simulink model "uz_mlp_three_layer"  (R2021a)
settings: Solver=FixedStepDiscrete  StartTime=0.0  StopTime=5000  RelTol=1e-3
values from neighbouring files (symbols this model uses):
  nn = nn.set_all_parameter(rand_variables)    [mlp2_definition.m]
  nn_data_type_max = 131071    [mlp2_definition.m]
  numInput = 13    [mlp2_definition.m]
  numOut = 4    [mlp2_definition.m]
libraries: hdlsllib x90, simulink x79, el_machinelearning x2
(part 3 of 4)

== system uz_mlp_three_layer/uz_mlp_three_layer/reluLayer_8Parallel/MAC7 ==
  rd_addr : Inport
  b : Inport  Port=2
  axi_signals : Inport  Port=3
  fromStateMachine : Inport  Port=4
  AND : Logic  IconShape=distinctive  AllPortsSameDT=off  OutDataTypeStr=boolean
  AND1 : Logic  IconShape=distinctive  AllPortsSameDT=off  OutDataTypeStr=boolean
  Bus Selector : BusSelector  OutputSignals=axi_weightData,axi_weightAddr,axi_weightsWriteEnable,axi_biasData,axi_biasAddr,axi_biasWriteEnable,axi_layerNr
  Bus Selector1 : BusSelector  OutputSignals=endin,validIn,startin,mac_counter,write_enable,n_perceptron
  Compare To Constant : simulink/Logic and Bit Operations/Compare To Constant  relop===  const=ParallelNr  OutDataTypeStr=boolean
  Compare To Constant1 : simulink/Logic and Bit Operations/Compare To Constant  relop===  const=ParallelNr  OutDataTypeStr=boolean
  Compare To Constant2 : simulink/Logic and Bit Operations/Compare To Constant  relop===  const=LayerNr  OutDataTypeStr=boolean
  Constant : Constant  Value=nStart  OutDataTypeStr=Inherit: Inherit via back propagation  SampleTime=-1
  Dual Port RAM System1 : hdlsllib/HDL RAMs/Dual Port RAM System  RAMType=Simple dual port  WriteOutputValue=New data  RAMInitialValue=[layer.bias(nStart:nEnd);zeros(1024-length(layer.bias(nStart:nEnd)),1)]  SimulateUsing=Code generation
      settings: SourceProductBaseCode=SL
  Dual Port RAM System2 : hdlsllib/HDL RAMs/Dual Port RAM System  RAMType=Simple dual port  WriteOutputValue=New data  RAMInitialValue=[0]  SimulateUsing=Code generation
      settings: SourceProductBaseCode=SL
  Dual Port RAM System3 : hdlsllib/HDL RAMs/Dual Port RAM System  RAMType=Simple dual port  WriteOutputValue=New data  RAMInitialValue=[0;reshape(layer.weights(:,nStart:nEnd),[],1);zeros(1023-length(reshape(layer.weights(:,nStart:nEnd),[],1)),1)]  SimulateUsing=Code generation
      settings: SourceProductBaseCode=SL
  Gain : Gain  Gain=size(layer.weights(:,nStart:nEnd),1)  OutDataTypeStr=Inherit: Same as input
  Multiply-Accumulate1 : hdlsllib/HDL Operations/Multiply-Accumulate  opMode=Streaming - using Start and End ports  initValueSetting=Dialog  initValue=0  initValueSetting2=Input port  initValue2=0  initValueSetting3=Dialog  initValue3=0  num_samples=2  RndMeth2=Floor  RndMeth3=Floor  datatype2=fixdt(1,32,14)  datatype3=Inherit: Inherit via back propagation  validOut=on  endInandOut=on  startOut=on  countOut=on  dim=-1  DoSatur=off  parallel=off
      settings: SourceProductBaseCode=SL
  Saturation1 : Saturate  UpperLimit=nn_data_type_max  LowerLimit=0
  Sum : Sum  Inputs=|++  OutDataTypeStr=Inherit: Same as first input
  Sum1 : Sum  Inputs=|++  OutDataTypeStr=Inherit: Same as first input
  Terminator : Terminator
  rd_dout : Outport
  startOut : Outport  Port=2
  endOut : Outport  Port=3
  wires:
  Dual Port RAM System1/1 -> Multiply-Accumulate1/6  "c"
  Saturation1/1 -> Dual Port RAM System2/1
  Multiply-Accumulate1/4 -> Terminator/1  "validout"
  Multiply-Accumulate1/2 -> startOut/1  "startout"
  Multiply-Accumulate1/1 -> Saturation1/1  "data"
  b/1 -> Multiply-Accumulate1/2
  Bus Selector1/6 -> Sum/1, Gain/1, Dual Port RAM System1/4  "<n_perceptron>"
  Constant/1 -> Sum/2
  Bus Selector1/1 -> Multiply-Accumulate1/4  "<endin>"
  Multiply-Accumulate1/3 -> endOut/1  "endout"
  Dual Port RAM System2/1 -> rd_dout/1
  Bus Selector1/4 -> Sum1/2  "<mac_counter>"
  Bus Selector1/2 -> Multiply-Accumulate1/5  "<validIn>"
  Bus Selector1/3 -> Multiply-Accumulate1/3  "<startin>"
  Gain/1 -> Sum1/1
  Sum1/1 -> Dual Port RAM System3/4
  Sum/1 -> Dual Port RAM System2/2
  Bus Selector1/5 -> Dual Port RAM System2/3  "<write_enable>"
  rd_addr/1 -> Dual Port RAM System2/4
  Dual Port RAM System3/1 -> Multiply-Accumulate1/1
  Bus Selector/4 -> Dual Port RAM System1/1  "<axi_biasData>"
  Bus Selector/5 -> Dual Port RAM System1/2  "<axi_biasAddr>"
  Bus Selector/6 -> Compare To Constant1/1  "<axi_biasWriteEnable>"
  Bus Selector/1 -> Dual Port RAM System3/1  "<axi_weightData>"
  Bus Selector/2 -> Dual Port RAM System3/2  "<axi_weightAddr>"
  Bus Selector/3 -> Compare To Constant/1  "<axi_weightsWriteEnable>"
  axi_signals/1 -> Bus Selector/1
  Compare To Constant/1 -> AND/1
  Compare To Constant1/1 -> AND1/1
  Compare To Constant2/1 -> AND1/2, AND/2
  AND/1 -> Dual Port RAM System3/3
  Bus Selector/7 -> Compare To Constant2/1  "<axi_layerNr>"
  AND1/1 -> Dual Port RAM System1/3
  fromStateMachine/1 -> Bus Selector1/1

== system uz_mlp_three_layer/uz_mlp_three_layer/reluLayer_8Parallel1/MAC ==
  rd_addr : Inport
  b : Inport  Port=2
  axi_signals : Inport  Port=3
  fromStateMachine : Inport  Port=4
  AND : Logic  IconShape=distinctive  AllPortsSameDT=off  OutDataTypeStr=boolean
  AND1 : Logic  IconShape=distinctive  AllPortsSameDT=off  OutDataTypeStr=boolean
  Bus Selector : BusSelector  OutputSignals=axi_weightData,axi_weightAddr,axi_weightsWriteEnable,axi_biasData,axi_biasAddr,axi_biasWriteEnable,axi_layerNr
  Bus Selector1 : BusSelector  OutputSignals=endin,validIn,startin,mac_counter,write_enable,n_perceptron
  Compare To Constant : simulink/Logic and Bit Operations/Compare To Constant  relop===  const=ParallelNr  OutDataTypeStr=boolean
  Compare To Constant1 : simulink/Logic and Bit Operations/Compare To Constant  relop===  const=ParallelNr  OutDataTypeStr=boolean
  Compare To Constant2 : simulink/Logic and Bit Operations/Compare To Constant  relop===  const=LayerNr  OutDataTypeStr=boolean
  Constant : Constant  Value=nStart  OutDataTypeStr=Inherit: Inherit via back propagation  SampleTime=-1
  Dual Port RAM System1 : hdlsllib/HDL RAMs/Dual Port RAM System  RAMType=Simple dual port  WriteOutputValue=New data  RAMInitialValue=[layer.bias(nStart:nEnd);zeros(1024-length(layer.bias(nStart:nEnd)),1)]  SimulateUsing=Code generation
      settings: SourceProductBaseCode=SL
  Dual Port RAM System2 : hdlsllib/HDL RAMs/Dual Port RAM System  RAMType=Simple dual port  WriteOutputValue=New data  RAMInitialValue=[0]  SimulateUsing=Code generation
      settings: SourceProductBaseCode=SL
  Dual Port RAM System3 : hdlsllib/HDL RAMs/Dual Port RAM System  RAMType=Simple dual port  WriteOutputValue=New data  RAMInitialValue=[0;reshape(layer.weights(:,nStart:nEnd),[],1);zeros(1023-length(reshape(layer.weights(:,nStart:nEnd),[],1)),1)]  SimulateUsing=Code generation
      settings: SourceProductBaseCode=SL
  Gain : Gain  Gain=size(layer.weights(:,nStart:nEnd),1)  OutDataTypeStr=Inherit: Same as input
  Multiply-Accumulate1 : hdlsllib/HDL Operations/Multiply-Accumulate  opMode=Streaming - using Start and End ports  initValueSetting=Dialog  initValue=0  initValueSetting2=Input port  initValue2=0  initValueSetting3=Dialog  initValue3=0  num_samples=2  RndMeth2=Floor  RndMeth3=Floor  datatype2=fixdt(1,32,14)  datatype3=Inherit: Inherit via back propagation  validOut=on  endInandOut=on  startOut=on  countOut=on  dim=-1  DoSatur=off  parallel=off
      settings: SourceProductBaseCode=SL
  Saturation1 : Saturate  UpperLimit=nn_data_type_max  LowerLimit=0
  Sum : Sum  Inputs=|++  OutDataTypeStr=Inherit: Same as first input
  Sum1 : Sum  Inputs=|++  OutDataTypeStr=Inherit: Same as first input
  Terminator : Terminator
  rd_dout : Outport
  startOut : Outport  Port=2
  endOut : Outport  Port=3
  wires:
  fromStateMachine/1 -> Bus Selector1/1
  AND1/1 -> Dual Port RAM System1/3
  Bus Selector/7 -> Compare To Constant2/1  "<axi_layerNr>"
  AND/1 -> Dual Port RAM System3/3
  Compare To Constant2/1 -> AND/2, AND1/2
  Compare To Constant1/1 -> AND1/1
  Compare To Constant/1 -> AND/1
  axi_signals/1 -> Bus Selector/1
  Bus Selector/3 -> Compare To Constant/1  "<axi_weightsWriteEnable>"
  Bus Selector/2 -> Dual Port RAM System3/2  "<axi_weightAddr>"
  Bus Selector/1 -> Dual Port RAM System3/1  "<axi_weightData>"
  Bus Selector/6 -> Compare To Constant1/1  "<axi_biasWriteEnable>"
  Bus Selector/5 -> Dual Port RAM System1/2  "<axi_biasAddr>"
  Bus Selector/4 -> Dual Port RAM System1/1  "<axi_biasData>"
  Dual Port RAM System3/1 -> Multiply-Accumulate1/1
  rd_addr/1 -> Dual Port RAM System2/4
  Bus Selector1/5 -> Dual Port RAM System2/3  "<write_enable>"
  Sum/1 -> Dual Port RAM System2/2
  Sum1/1 -> Dual Port RAM System3/4
  Gain/1 -> Sum1/1
  Bus Selector1/3 -> Multiply-Accumulate1/3  "<startin>"
  Bus Selector1/2 -> Multiply-Accumulate1/5  "<validIn>"
  Bus Selector1/4 -> Sum1/2  "<mac_counter>"
  Dual Port RAM System2/1 -> rd_dout/1
  Multiply-Accumulate1/3 -> endOut/1  "endout"
  Bus Selector1/1 -> Multiply-Accumulate1/4  "<endin>"
  Constant/1 -> Sum/2
  Bus Selector1/6 -> Dual Port RAM System1/4, Gain/1, Sum/1  "<n_perceptron>"
  b/1 -> Multiply-Accumulate1/2
  Multiply-Accumulate1/1 -> Saturation1/1  "data"
  Multiply-Accumulate1/2 -> startOut/1  "startout"
  Multiply-Accumulate1/4 -> Terminator/1  "validout"
  Saturation1/1 -> Dual Port RAM System2/1
  Dual Port RAM System1/1 -> Multiply-Accumulate1/6  "c"

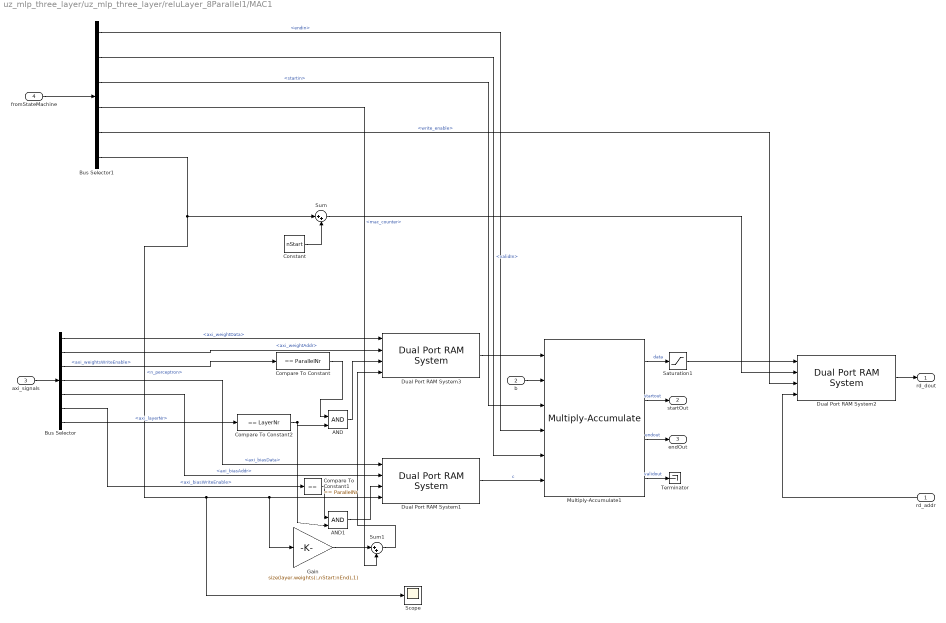
== system uz_mlp_three_layer/uz_mlp_three_layer/reluLayer_8Parallel1/MAC1 ==
  rd_addr : Inport
  b : Inport  Port=2
  axi_signals : Inport  Port=3
  fromStateMachine : Inport  Port=4
  AND : Logic  IconShape=distinctive  AllPortsSameDT=off  OutDataTypeStr=boolean
  AND1 : Logic  IconShape=distinctive  AllPortsSameDT=off  OutDataTypeStr=boolean
  Bus Selector : BusSelector  OutputSignals=axi_weightData,axi_weightAddr,axi_weightsWriteEnable,axi_biasData,axi_biasAddr,axi_biasWriteEnable,axi_layerNr
  Bus Selector1 : BusSelector  OutputSignals=endin,validIn,startin,mac_counter,write_enable,n_perceptron
  Compare To Constant : simulink/Logic and Bit Operations/Compare To Constant  relop===  const=ParallelNr  OutDataTypeStr=boolean
  Compare To Constant1 : simulink/Logic and Bit Operations/Compare To Constant  relop===  const=ParallelNr  OutDataTypeStr=boolean
  Compare To Constant2 : simulink/Logic and Bit Operations/Compare To Constant  relop===  const=LayerNr  OutDataTypeStr=boolean
  Constant : Constant  Value=nStart  OutDataTypeStr=Inherit: Inherit via back propagation  SampleTime=-1
  Dual Port RAM System1 : hdlsllib/HDL RAMs/Dual Port RAM System  RAMType=Simple dual port  WriteOutputValue=New data  RAMInitialValue=[layer.bias(nStart:nEnd);zeros(1024-length(layer.bias(nStart:nEnd)),1)]  SimulateUsing=Code generation
      settings: SourceProductBaseCode=SL
  Dual Port RAM System2 : hdlsllib/HDL RAMs/Dual Port RAM System  RAMType=Simple dual port  WriteOutputValue=New data  RAMInitialValue=[0]  SimulateUsing=Code generation
      settings: SourceProductBaseCode=SL
  Dual Port RAM System3 : hdlsllib/HDL RAMs/Dual Port RAM System  RAMType=Simple dual port  WriteOutputValue=New data  RAMInitialValue=[0;reshape(layer.weights(:,nStart:nEnd),[],1);zeros(1023-length(reshape(layer.weights(:,nStart:nEnd),[],1)),1)]  SimulateUsing=Code generation
      settings: SourceProductBaseCode=SL
  Gain : Gain  Gain=size(layer.weights(:,nStart:nEnd),1)  OutDataTypeStr=Inherit: Same as input
  Multiply-Accumulate1 : hdlsllib/HDL Operations/Multiply-Accumulate  opMode=Streaming - using Start and End ports  initValueSetting=Dialog  initValue=0  initValueSetting2=Input port  initValue2=0  initValueSetting3=Dialog  initValue3=0  num_samples=2  RndMeth2=Floor  RndMeth3=Floor  datatype2=fixdt(1,32,14)  datatype3=Inherit: Inherit via back propagation  validOut=on  endInandOut=on  startOut=on  countOut=on  dim=-1  DoSatur=off  parallel=off
      settings: SourceProductBaseCode=SL
  Saturation1 : Saturate  UpperLimit=nn_data_type_max  LowerLimit=0
  Scope : Scope
  Sum : Sum  Inputs=|++  OutDataTypeStr=Inherit: Same as first input
  Sum1 : Sum  Inputs=|++  OutDataTypeStr=Inherit: Same as first input
  Terminator : Terminator
  rd_dout : Outport
  startOut : Outport  Port=2
  endOut : Outport  Port=3
  wires:
  fromStateMachine/1 -> Bus Selector1/1
  AND1/1 -> Dual Port RAM System1/3
  Bus Selector/7 -> Compare To Constant2/1  "<axi_layerNr>"
  AND/1 -> Dual Port RAM System3/3
  Compare To Constant2/1 -> AND/2, AND1/2
  Compare To Constant1/1 -> AND1/1
  Compare To Constant/1 -> AND/1
  axi_signals/1 -> Bus Selector/1
  Bus Selector/3 -> Compare To Constant/1  "<axi_weightsWriteEnable>"
  Bus Selector/2 -> Dual Port RAM System3/2  "<axi_weightAddr>"
  Bus Selector/1 -> Dual Port RAM System3/1  "<axi_weightData>"
  Bus Selector/6 -> Compare To Constant1/1  "<axi_biasWriteEnable>"
  Bus Selector/5 -> Dual Port RAM System1/2  "<axi_biasAddr>"
  Bus Selector/4 -> Dual Port RAM System1/1  "<axi_biasData>"
  Dual Port RAM System3/1 -> Multiply-Accumulate1/1
  rd_addr/1 -> Dual Port RAM System2/4
  Bus Selector1/5 -> Dual Port RAM System2/3  "<write_enable>"
  Sum/1 -> Dual Port RAM System2/2
  Sum1/1 -> Dual Port RAM System3/4
  Gain/1 -> Sum1/1
  Bus Selector1/3 -> Multiply-Accumulate1/3  "<startin>"
  Bus Selector1/2 -> Multiply-Accumulate1/5  "<validIn>"
  Bus Selector1/4 -> Sum1/2  "<mac_counter>"
  Dual Port RAM System2/1 -> rd_dout/1
  Multiply-Accumulate1/3 -> endOut/1  "endout"
  Bus Selector1/1 -> Multiply-Accumulate1/4  "<endin>"
  Constant/1 -> Sum/2
  Bus Selector1/6 -> Scope/1, Dual Port RAM System1/4, Gain/1, Sum/1  "<n_perceptron>"
  b/1 -> Multiply-Accumulate1/2
  Multiply-Accumulate1/1 -> Saturation1/1  "data"
  Multiply-Accumulate1/2 -> startOut/1  "startout"
  Multiply-Accumulate1/4 -> Terminator/1  "validout"
  Saturation1/1 -> Dual Port RAM System2/1
  Dual Port RAM System1/1 -> Multiply-Accumulate1/6  "c"

== system uz_mlp_three_layer/uz_mlp_three_layer/reluLayer_8Parallel1/MAC3 ==
  rd_addr : Inport
  b : Inport  Port=2
  axi_signals : Inport  Port=3
  fromStateMachine : Inport  Port=4
  AND : Logic  IconShape=distinctive  AllPortsSameDT=off  OutDataTypeStr=boolean
  AND1 : Logic  IconShape=distinctive  AllPortsSameDT=off  OutDataTypeStr=boolean
  Bus Selector : BusSelector  OutputSignals=axi_weightData,axi_weightAddr,axi_weightsWriteEnable,axi_biasData,axi_biasAddr,axi_biasWriteEnable,axi_layerNr
  Bus Selector1 : BusSelector  OutputSignals=endin,validIn,startin,mac_counter,write_enable,n_perceptron
  Compare To Constant : simulink/Logic and Bit Operations/Compare To Constant  relop===  const=ParallelNr  OutDataTypeStr=boolean
  Compare To Constant1 : simulink/Logic and Bit Operations/Compare To Constant  relop===  const=ParallelNr  OutDataTypeStr=boolean
  Compare To Constant2 : simulink/Logic and Bit Operations/Compare To Constant  relop===  const=LayerNr  OutDataTypeStr=boolean
  Constant : Constant  Value=nStart  OutDataTypeStr=Inherit: Inherit via back propagation  SampleTime=-1
  Dual Port RAM System1 : hdlsllib/HDL RAMs/Dual Port RAM System  RAMType=Simple dual port  WriteOutputValue=New data  RAMInitialValue=[layer.bias(nStart:nEnd);zeros(1024-length(layer.bias(nStart:nEnd)),1)]  SimulateUsing=Code generation
      settings: SourceProductBaseCode=SL
  Dual Port RAM System2 : hdlsllib/HDL RAMs/Dual Port RAM System  RAMType=Simple dual port  WriteOutputValue=New data  RAMInitialValue=[0]  SimulateUsing=Code generation
      settings: SourceProductBaseCode=SL
  Dual Port RAM System3 : hdlsllib/HDL RAMs/Dual Port RAM System  RAMType=Simple dual port  WriteOutputValue=New data  RAMInitialValue=[0;reshape(layer.weights(:,nStart:nEnd),[],1);zeros(1023-length(reshape(layer.weights(:,nStart:nEnd),[],1)),1)]  SimulateUsing=Code generation
      settings: SourceProductBaseCode=SL
  Gain : Gain  Gain=size(layer.weights(:,nStart:nEnd),1)  OutDataTypeStr=Inherit: Same as input
  Multiply-Accumulate1 : hdlsllib/HDL Operations/Multiply-Accumulate  opMode=Streaming - using Start and End ports  initValueSetting=Dialog  initValue=0  initValueSetting2=Input port  initValue2=0  initValueSetting3=Dialog  initValue3=0  num_samples=2  RndMeth2=Floor  RndMeth3=Floor  datatype2=fixdt(1,32,14)  datatype3=Inherit: Inherit via back propagation  validOut=on  endInandOut=on  startOut=on  countOut=on  dim=-1  DoSatur=off  parallel=off
      settings: SourceProductBaseCode=SL
  Saturation1 : Saturate  UpperLimit=nn_data_type_max  LowerLimit=0
  Sum : Sum  Inputs=|++  OutDataTypeStr=Inherit: Same as first input
  Sum1 : Sum  Inputs=|++  OutDataTypeStr=Inherit: Same as first input
  Terminator : Terminator
  rd_dout : Outport
  startOut : Outport  Port=2
  endOut : Outport  Port=3
  wires:
  fromStateMachine/1 -> Bus Selector1/1
  AND1/1 -> Dual Port RAM System1/3
  Bus Selector/7 -> Compare To Constant2/1  "<axi_layerNr>"
  AND/1 -> Dual Port RAM System3/3
  Compare To Constant2/1 -> AND/2, AND1/2
  Compare To Constant1/1 -> AND1/1
  Compare To Constant/1 -> AND/1
  axi_signals/1 -> Bus Selector/1
  Bus Selector/3 -> Compare To Constant/1  "<axi_weightsWriteEnable>"
  Bus Selector/2 -> Dual Port RAM System3/2  "<axi_weightAddr>"
  Bus Selector/1 -> Dual Port RAM System3/1  "<axi_weightData>"
  Bus Selector/6 -> Compare To Constant1/1  "<axi_biasWriteEnable>"
  Bus Selector/5 -> Dual Port RAM System1/2  "<axi_biasAddr>"
  Bus Selector/4 -> Dual Port RAM System1/1  "<axi_biasData>"
  Dual Port RAM System3/1 -> Multiply-Accumulate1/1
  rd_addr/1 -> Dual Port RAM System2/4
  Bus Selector1/5 -> Dual Port RAM System2/3  "<write_enable>"
  Sum/1 -> Dual Port RAM System2/2
  Sum1/1 -> Dual Port RAM System3/4
  Gain/1 -> Sum1/1
  Bus Selector1/3 -> Multiply-Accumulate1/3  "<startin>"
  Bus Selector1/2 -> Multiply-Accumulate1/5  "<validIn>"
  Bus Selector1/4 -> Sum1/2  "<mac_counter>"
  Dual Port RAM System2/1 -> rd_dout/1
  Multiply-Accumulate1/3 -> endOut/1  "endout"
  Bus Selector1/1 -> Multiply-Accumulate1/4  "<endin>"
  Constant/1 -> Sum/2
  Bus Selector1/6 -> Dual Port RAM System1/4, Gain/1, Sum/1  "<n_perceptron>"
  b/1 -> Multiply-Accumulate1/2
  Multiply-Accumulate1/1 -> Saturation1/1  "data"
  Multiply-Accumulate1/2 -> startOut/1  "startout"
  Multiply-Accumulate1/4 -> Terminator/1  "validout"
  Saturation1/1 -> Dual Port RAM System2/1
  Dual Port RAM System1/1 -> Multiply-Accumulate1/6  "c"

== system uz_mlp_three_layer/uz_mlp_three_layer/reluLayer_8Parallel1/MAC4 ==
  rd_addr : Inport
  b : Inport  Port=2
  axi_signals : Inport  Port=3
  fromStateMachine : Inport  Port=4
  AND : Logic  IconShape=distinctive  AllPortsSameDT=off  OutDataTypeStr=boolean
  AND1 : Logic  IconShape=distinctive  AllPortsSameDT=off  OutDataTypeStr=boolean
  Bus Selector : BusSelector  OutputSignals=axi_weightData,axi_weightAddr,axi_weightsWriteEnable,axi_biasData,axi_biasAddr,axi_biasWriteEnable,axi_layerNr
  Bus Selector1 : BusSelector  OutputSignals=endin,validIn,startin,mac_counter,write_enable,n_perceptron
  Compare To Constant : simulink/Logic and Bit Operations/Compare To Constant  relop===  const=ParallelNr  OutDataTypeStr=boolean
  Compare To Constant1 : simulink/Logic and Bit Operations/Compare To Constant  relop===  const=ParallelNr  OutDataTypeStr=boolean
  Compare To Constant2 : simulink/Logic and Bit Operations/Compare To Constant  relop===  const=LayerNr  OutDataTypeStr=boolean
  Constant : Constant  Value=nStart  OutDataTypeStr=Inherit: Inherit via back propagation  SampleTime=-1
  Dual Port RAM System1 : hdlsllib/HDL RAMs/Dual Port RAM System  RAMType=Simple dual port  WriteOutputValue=New data  RAMInitialValue=[layer.bias(nStart:nEnd);zeros(1024-length(layer.bias(nStart:nEnd)),1)]  SimulateUsing=Code generation
      settings: SourceProductBaseCode=SL
  Dual Port RAM System2 : hdlsllib/HDL RAMs/Dual Port RAM System  RAMType=Simple dual port  WriteOutputValue=New data  RAMInitialValue=[0]  SimulateUsing=Code generation
      settings: SourceProductBaseCode=SL
  Dual Port RAM System3 : hdlsllib/HDL RAMs/Dual Port RAM System  RAMType=Simple dual port  WriteOutputValue=New data  RAMInitialValue=[0;reshape(layer.weights(:,nStart:nEnd),[],1);zeros(1023-length(reshape(layer.weights(:,nStart:nEnd),[],1)),1)]  SimulateUsing=Code generation
      settings: SourceProductBaseCode=SL
  Gain : Gain  Gain=size(layer.weights(:,nStart:nEnd),1)  OutDataTypeStr=Inherit: Same as input
  Multiply-Accumulate1 : hdlsllib/HDL Operations/Multiply-Accumulate  opMode=Streaming - using Start and End ports  initValueSetting=Dialog  initValue=0  initValueSetting2=Input port  initValue2=0  initValueSetting3=Dialog  initValue3=0  num_samples=2  RndMeth2=Floor  RndMeth3=Floor  datatype2=fixdt(1,32,14)  datatype3=Inherit: Inherit via back propagation  validOut=on  endInandOut=on  startOut=on  countOut=on  dim=-1  DoSatur=off  parallel=off
      settings: SourceProductBaseCode=SL
  Saturation1 : Saturate  UpperLimit=nn_data_type_max  LowerLimit=0
  Sum : Sum  Inputs=|++  OutDataTypeStr=Inherit: Same as first input
  Sum1 : Sum  Inputs=|++  OutDataTypeStr=Inherit: Same as first input
  Terminator : Terminator
  rd_dout : Outport
  startOut : Outport  Port=2
  endOut : Outport  Port=3
  wires:
  fromStateMachine/1 -> Bus Selector1/1
  AND1/1 -> Dual Port RAM System1/3
  Bus Selector/7 -> Compare To Constant2/1  "<axi_layerNr>"
  AND/1 -> Dual Port RAM System3/3
  Compare To Constant2/1 -> AND/2, AND1/2
  Compare To Constant1/1 -> AND1/1
  Compare To Constant/1 -> AND/1
  axi_signals/1 -> Bus Selector/1
  Bus Selector/3 -> Compare To Constant/1  "<axi_weightsWriteEnable>"
  Bus Selector/2 -> Dual Port RAM System3/2  "<axi_weightAddr>"
  Bus Selector/1 -> Dual Port RAM System3/1  "<axi_weightData>"
  Bus Selector/6 -> Compare To Constant1/1  "<axi_biasWriteEnable>"
  Bus Selector/5 -> Dual Port RAM System1/2  "<axi_biasAddr>"
  Bus Selector/4 -> Dual Port RAM System1/1  "<axi_biasData>"
  Dual Port RAM System3/1 -> Multiply-Accumulate1/1
  rd_addr/1 -> Dual Port RAM System2/4
  Bus Selector1/5 -> Dual Port RAM System2/3  "<write_enable>"
  Sum/1 -> Dual Port RAM System2/2
  Sum1/1 -> Dual Port RAM System3/4
  Gain/1 -> Sum1/1
  Bus Selector1/3 -> Multiply-Accumulate1/3  "<startin>"
  Bus Selector1/2 -> Multiply-Accumulate1/5  "<validIn>"
  Bus Selector1/4 -> Sum1/2  "<mac_counter>"
  Dual Port RAM System2/1 -> rd_dout/1
  Multiply-Accumulate1/3 -> endOut/1  "endout"
  Bus Selector1/1 -> Multiply-Accumulate1/4  "<endin>"
  Constant/1 -> Sum/2
  Bus Selector1/6 -> Dual Port RAM System1/4, Gain/1, Sum/1  "<n_perceptron>"
  b/1 -> Multiply-Accumulate1/2
  Multiply-Accumulate1/1 -> Saturation1/1  "data"
  Multiply-Accumulate1/2 -> startOut/1  "startout"
  Multiply-Accumulate1/4 -> Terminator/1  "validout"
  Saturation1/1 -> Dual Port RAM System2/1
  Dual Port RAM System1/1 -> Multiply-Accumulate1/6  "c"

== system uz_mlp_three_layer/uz_mlp_three_layer/reluLayer_8Parallel1/MAC5 ==
  rd_addr : Inport
  b : Inport  Port=2
  axi_signals : Inport  Port=3
  fromStateMachine : Inport  Port=4
  AND : Logic  IconShape=distinctive  AllPortsSameDT=off  OutDataTypeStr=boolean
  AND1 : Logic  IconShape=distinctive  AllPortsSameDT=off  OutDataTypeStr=boolean
  Bus Selector : BusSelector  OutputSignals=axi_weightData,axi_weightAddr,axi_weightsWriteEnable,axi_biasData,axi_biasAddr,axi_biasWriteEnable,axi_layerNr
  Bus Selector1 : BusSelector  OutputSignals=endin,validIn,startin,mac_counter,write_enable,n_perceptron
  Compare To Constant : simulink/Logic and Bit Operations/Compare To Constant  relop===  const=ParallelNr  OutDataTypeStr=boolean
  Compare To Constant1 : simulink/Logic and Bit Operations/Compare To Constant  relop===  const=ParallelNr  OutDataTypeStr=boolean
  Compare To Constant2 : simulink/Logic and Bit Operations/Compare To Constant  relop===  const=LayerNr  OutDataTypeStr=boolean
  Constant : Constant  Value=nStart  OutDataTypeStr=Inherit: Inherit via back propagation  SampleTime=-1
  Dual Port RAM System1 : hdlsllib/HDL RAMs/Dual Port RAM System  RAMType=Simple dual port  WriteOutputValue=New data  RAMInitialValue=[layer.bias(nStart:nEnd);zeros(1024-length(layer.bias(nStart:nEnd)),1)]  SimulateUsing=Code generation
      settings: SourceProductBaseCode=SL
  Dual Port RAM System2 : hdlsllib/HDL RAMs/Dual Port RAM System  RAMType=Simple dual port  WriteOutputValue=New data  RAMInitialValue=[0]  SimulateUsing=Code generation
      settings: SourceProductBaseCode=SL
  Dual Port RAM System3 : hdlsllib/HDL RAMs/Dual Port RAM System  RAMType=Simple dual port  WriteOutputValue=New data  RAMInitialValue=[0;reshape(layer.weights(:,nStart:nEnd),[],1);zeros(1023-length(reshape(layer.weights(:,nStart:nEnd),[],1)),1)]  SimulateUsing=Code generation
      settings: SourceProductBaseCode=SL
  Gain : Gain  Gain=size(layer.weights(:,nStart:nEnd),1)  OutDataTypeStr=Inherit: Same as input
  Multiply-Accumulate1 : hdlsllib/HDL Operations/Multiply-Accumulate  opMode=Streaming - using Start and End ports  initValueSetting=Dialog  initValue=0  initValueSetting2=Input port  initValue2=0  initValueSetting3=Dialog  initValue3=0  num_samples=2  RndMeth2=Floor  RndMeth3=Floor  datatype2=fixdt(1,32,14)  datatype3=Inherit: Inherit via back propagation  validOut=on  endInandOut=on  startOut=on  countOut=on  dim=-1  DoSatur=off  parallel=off
      settings: SourceProductBaseCode=SL
  Saturation1 : Saturate  UpperLimit=nn_data_type_max  LowerLimit=0
  Sum : Sum  Inputs=|++  OutDataTypeStr=Inherit: Same as first input
  Sum1 : Sum  Inputs=|++  OutDataTypeStr=Inherit: Same as first input
  Terminator : Terminator
  rd_dout : Outport
  startOut : Outport  Port=2
  endOut : Outport  Port=3
  wires:
  fromStateMachine/1 -> Bus Selector1/1
  AND1/1 -> Dual Port RAM System1/3
  Bus Selector/7 -> Compare To Constant2/1  "<axi_layerNr>"
  AND/1 -> Dual Port RAM System3/3
  Compare To Constant2/1 -> AND/2, AND1/2
  Compare To Constant1/1 -> AND1/1
  Compare To Constant/1 -> AND/1
  axi_signals/1 -> Bus Selector/1
  Bus Selector/3 -> Compare To Constant/1  "<axi_weightsWriteEnable>"
  Bus Selector/2 -> Dual Port RAM System3/2  "<axi_weightAddr>"
  Bus Selector/1 -> Dual Port RAM System3/1  "<axi_weightData>"
  Bus Selector/6 -> Compare To Constant1/1  "<axi_biasWriteEnable>"
  Bus Selector/5 -> Dual Port RAM System1/2  "<axi_biasAddr>"
  Bus Selector/4 -> Dual Port RAM System1/1  "<axi_biasData>"
  Dual Port RAM System3/1 -> Multiply-Accumulate1/1
  rd_addr/1 -> Dual Port RAM System2/4
  Bus Selector1/5 -> Dual Port RAM System2/3  "<write_enable>"
  Sum/1 -> Dual Port RAM System2/2
  Sum1/1 -> Dual Port RAM System3/4
  Gain/1 -> Sum1/1
  Bus Selector1/3 -> Multiply-Accumulate1/3  "<startin>"
  Bus Selector1/2 -> Multiply-Accumulate1/5  "<validIn>"
  Bus Selector1/4 -> Sum1/2  "<mac_counter>"
  Dual Port RAM System2/1 -> rd_dout/1
  Multiply-Accumulate1/3 -> endOut/1  "endout"
  Bus Selector1/1 -> Multiply-Accumulate1/4  "<endin>"
  Constant/1 -> Sum/2
  Bus Selector1/6 -> Dual Port RAM System1/4, Gain/1, Sum/1  "<n_perceptron>"
  b/1 -> Multiply-Accumulate1/2
  Multiply-Accumulate1/1 -> Saturation1/1  "data"
  Multiply-Accumulate1/2 -> startOut/1  "startout"
  Multiply-Accumulate1/4 -> Terminator/1  "validout"
  Saturation1/1 -> Dual Port RAM System2/1
  Dual Port RAM System1/1 -> Multiply-Accumulate1/6  "c"

== system uz_mlp_three_layer/uz_mlp_three_layer/reluLayer_8Parallel1/MAC6 ==
  rd_addr : Inport
  b : Inport  Port=2
  axi_signals : Inport  Port=3
  fromStateMachine : Inport  Port=4
  AND : Logic  IconShape=distinctive  AllPortsSameDT=off  OutDataTypeStr=boolean
  AND1 : Logic  IconShape=distinctive  AllPortsSameDT=off  OutDataTypeStr=boolean
  Bus Selector : BusSelector  OutputSignals=axi_weightData,axi_weightAddr,axi_weightsWriteEnable,axi_biasData,axi_biasAddr,axi_biasWriteEnable,axi_layerNr
  Bus Selector1 : BusSelector  OutputSignals=endin,validIn,startin,mac_counter,write_enable,n_perceptron
  Compare To Constant : simulink/Logic and Bit Operations/Compare To Constant  relop===  const=ParallelNr  OutDataTypeStr=boolean
  Compare To Constant1 : simulink/Logic and Bit Operations/Compare To Constant  relop===  const=ParallelNr  OutDataTypeStr=boolean
  Compare To Constant2 : simulink/Logic and Bit Operations/Compare To Constant  relop===  const=LayerNr  OutDataTypeStr=boolean
  Constant : Constant  Value=nStart  OutDataTypeStr=Inherit: Inherit via back propagation  SampleTime=-1
  Dual Port RAM System1 : hdlsllib/HDL RAMs/Dual Port RAM System  RAMType=Simple dual port  WriteOutputValue=New data  RAMInitialValue=[layer.bias(nStart:nEnd);zeros(1024-length(layer.bias(nStart:nEnd)),1)]  SimulateUsing=Code generation
      settings: SourceProductBaseCode=SL
  Dual Port RAM System2 : hdlsllib/HDL RAMs/Dual Port RAM System  RAMType=Simple dual port  WriteOutputValue=New data  RAMInitialValue=[0]  SimulateUsing=Code generation
      settings: SourceProductBaseCode=SL
  Dual Port RAM System3 : hdlsllib/HDL RAMs/Dual Port RAM System  RAMType=Simple dual port  WriteOutputValue=New data  RAMInitialValue=[0;reshape(layer.weights(:,nStart:nEnd),[],1);zeros(1023-length(reshape(layer.weights(:,nStart:nEnd),[],1)),1)]  SimulateUsing=Code generation
      settings: SourceProductBaseCode=SL
  Gain : Gain  Gain=size(layer.weights(:,nStart:nEnd),1)  OutDataTypeStr=Inherit: Same as input
  Multiply-Accumulate1 : hdlsllib/HDL Operations/Multiply-Accumulate  opMode=Streaming - using Start and End ports  initValueSetting=Dialog  initValue=0  initValueSetting2=Input port  initValue2=0  initValueSetting3=Dialog  initValue3=0  num_samples=2  RndMeth2=Floor  RndMeth3=Floor  datatype2=fixdt(1,32,14)  datatype3=Inherit: Inherit via back propagation  validOut=on  endInandOut=on  startOut=on  countOut=on  dim=-1  DoSatur=off  parallel=off
      settings: SourceProductBaseCode=SL
  Saturation1 : Saturate  UpperLimit=nn_data_type_max  LowerLimit=0
  Sum : Sum  Inputs=|++  OutDataTypeStr=Inherit: Same as first input
  Sum1 : Sum  Inputs=|++  OutDataTypeStr=Inherit: Same as first input
  Terminator : Terminator
  rd_dout : Outport
  startOut : Outport  Port=2
  endOut : Outport  Port=3
  wires:
  fromStateMachine/1 -> Bus Selector1/1
  AND1/1 -> Dual Port RAM System1/3
  Bus Selector/7 -> Compare To Constant2/1  "<axi_layerNr>"
  AND/1 -> Dual Port RAM System3/3
  Compare To Constant2/1 -> AND/2, AND1/2
  Compare To Constant1/1 -> AND1/1
  Compare To Constant/1 -> AND/1
  axi_signals/1 -> Bus Selector/1
  Bus Selector/3 -> Compare To Constant/1  "<axi_weightsWriteEnable>"
  Bus Selector/2 -> Dual Port RAM System3/2  "<axi_weightAddr>"
  Bus Selector/1 -> Dual Port RAM System3/1  "<axi_weightData>"
  Bus Selector/6 -> Compare To Constant1/1  "<axi_biasWriteEnable>"
  Bus Selector/5 -> Dual Port RAM System1/2  "<axi_biasAddr>"
  Bus Selector/4 -> Dual Port RAM System1/1  "<axi_biasData>"
  Dual Port RAM System3/1 -> Multiply-Accumulate1/1
  rd_addr/1 -> Dual Port RAM System2/4
  Bus Selector1/5 -> Dual Port RAM System2/3  "<write_enable>"
  Sum/1 -> Dual Port RAM System2/2
  Sum1/1 -> Dual Port RAM System3/4
  Gain/1 -> Sum1/1
  Bus Selector1/3 -> Multiply-Accumulate1/3  "<startin>"
  Bus Selector1/2 -> Multiply-Accumulate1/5  "<validIn>"
  Bus Selector1/4 -> Sum1/2  "<mac_counter>"
  Dual Port RAM System2/1 -> rd_dout/1
  Multiply-Accumulate1/3 -> endOut/1  "endout"
  Bus Selector1/1 -> Multiply-Accumulate1/4  "<endin>"
  Constant/1 -> Sum/2
  Bus Selector1/6 -> Dual Port RAM System1/4, Gain/1, Sum/1  "<n_perceptron>"
  b/1 -> Multiply-Accumulate1/2
  Multiply-Accumulate1/1 -> Saturation1/1  "data"
  Multiply-Accumulate1/2 -> startOut/1  "startout"
  Multiply-Accumulate1/4 -> Terminator/1  "validout"
  Saturation1/1 -> Dual Port RAM System2/1
  Dual Port RAM System1/1 -> Multiply-Accumulate1/6  "c"

== system uz_mlp_three_layer/uz_mlp_three_layer/reluLayer_8Parallel1/MAC7 ==
  rd_addr : Inport
  b : Inport  Port=2
  axi_signals : Inport  Port=3
  fromStateMachine : Inport  Port=4
  AND : Logic  IconShape=distinctive  AllPortsSameDT=off  OutDataTypeStr=boolean
  AND1 : Logic  IconShape=distinctive  AllPortsSameDT=off  OutDataTypeStr=boolean
  Bus Selector : BusSelector  OutputSignals=axi_weightData,axi_weightAddr,axi_weightsWriteEnable,axi_biasData,axi_biasAddr,axi_biasWriteEnable,axi_layerNr
  Bus Selector1 : BusSelector  OutputSignals=endin,validIn,startin,mac_counter,write_enable,n_perceptron
  Compare To Constant : simulink/Logic and Bit Operations/Compare To Constant  relop===  const=ParallelNr  OutDataTypeStr=boolean
  Compare To Constant1 : simulink/Logic and Bit Operations/Compare To Constant  relop===  const=ParallelNr  OutDataTypeStr=boolean
  Compare To Constant2 : simulink/Logic and Bit Operations/Compare To Constant  relop===  const=LayerNr  OutDataTypeStr=boolean
  Constant : Constant  Value=nStart  OutDataTypeStr=Inherit: Inherit via back propagation  SampleTime=-1
  Dual Port RAM System1 : hdlsllib/HDL RAMs/Dual Port RAM System  RAMType=Simple dual port  WriteOutputValue=New data  RAMInitialValue=[layer.bias(nStart:nEnd);zeros(1024-length(layer.bias(nStart:nEnd)),1)]  SimulateUsing=Code generation
      settings: SourceProductBaseCode=SL
  Dual Port RAM System2 : hdlsllib/HDL RAMs/Dual Port RAM System  RAMType=Simple dual port  WriteOutputValue=New data  RAMInitialValue=[0]  SimulateUsing=Code generation
      settings: SourceProductBaseCode=SL
  Dual Port RAM System3 : hdlsllib/HDL RAMs/Dual Port RAM System  RAMType=Simple dual port  WriteOutputValue=New data  RAMInitialValue=[0;reshape(layer.weights(:,nStart:nEnd),[],1);zeros(1023-length(reshape(layer.weights(:,nStart:nEnd),[],1)),1)]  SimulateUsing=Code generation
      settings: SourceProductBaseCode=SL
  Gain : Gain  Gain=size(layer.weights(:,nStart:nEnd),1)  OutDataTypeStr=Inherit: Same as input
  Multiply-Accumulate1 : hdlsllib/HDL Operations/Multiply-Accumulate  opMode=Streaming - using Start and End ports  initValueSetting=Dialog  initValue=0  initValueSetting2=Input port  initValue2=0  initValueSetting3=Dialog  initValue3=0  num_samples=2  RndMeth2=Floor  RndMeth3=Floor  datatype2=fixdt(1,32,14)  datatype3=Inherit: Inherit via back propagation  validOut=on  endInandOut=on  startOut=on  countOut=on  dim=-1  DoSatur=off  parallel=off
      settings: SourceProductBaseCode=SL
  Saturation1 : Saturate  UpperLimit=nn_data_type_max  LowerLimit=0
  Sum : Sum  Inputs=|++  OutDataTypeStr=Inherit: Same as first input
  Sum1 : Sum  Inputs=|++  OutDataTypeStr=Inherit: Same as first input
  Terminator : Terminator
  rd_dout : Outport
  startOut : Outport  Port=2
  endOut : Outport  Port=3
  wires:
  fromStateMachine/1 -> Bus Selector1/1
  AND1/1 -> Dual Port RAM System1/3
  Bus Selector/7 -> Compare To Constant2/1  "<axi_layerNr>"
  AND/1 -> Dual Port RAM System3/3
  Compare To Constant2/1 -> AND/2, AND1/2
  Compare To Constant1/1 -> AND1/1
  Compare To Constant/1 -> AND/1
  axi_signals/1 -> Bus Selector/1
  Bus Selector/3 -> Compare To Constant/1  "<axi_weightsWriteEnable>"
  Bus Selector/2 -> Dual Port RAM System3/2  "<axi_weightAddr>"
  Bus Selector/1 -> Dual Port RAM System3/1  "<axi_weightData>"
  Bus Selector/6 -> Compare To Constant1/1  "<axi_biasWriteEnable>"
  Bus Selector/5 -> Dual Port RAM System1/2  "<axi_biasAddr>"
  Bus Selector/4 -> Dual Port RAM System1/1  "<axi_biasData>"
  Dual Port RAM System3/1 -> Multiply-Accumulate1/1
  rd_addr/1 -> Dual Port RAM System2/4
  Bus Selector1/5 -> Dual Port RAM System2/3  "<write_enable>"
  Sum/1 -> Dual Port RAM System2/2
  Sum1/1 -> Dual Port RAM System3/4
  Gain/1 -> Sum1/1
  Bus Selector1/3 -> Multiply-Accumulate1/3  "<startin>"
  Bus Selector1/2 -> Multiply-Accumulate1/5  "<validIn>"
  Bus Selector1/4 -> Sum1/2  "<mac_counter>"
  Dual Port RAM System2/1 -> rd_dout/1
  Multiply-Accumulate1/3 -> endOut/1  "endout"
  Bus Selector1/1 -> Multiply-Accumulate1/4  "<endin>"
  Constant/1 -> Sum/2
  Bus Selector1/6 -> Dual Port RAM System1/4, Gain/1, Sum/1  "<n_perceptron>"
  b/1 -> Multiply-Accumulate1/2
  Multiply-Accumulate1/1 -> Saturation1/1  "data"
  Multiply-Accumulate1/2 -> startOut/1  "startout"
  Multiply-Accumulate1/4 -> Terminator/1  "validout"
  Saturation1/1 -> Dual Port RAM System2/1
  Dual Port RAM System1/1 -> Multiply-Accumulate1/6  "c"

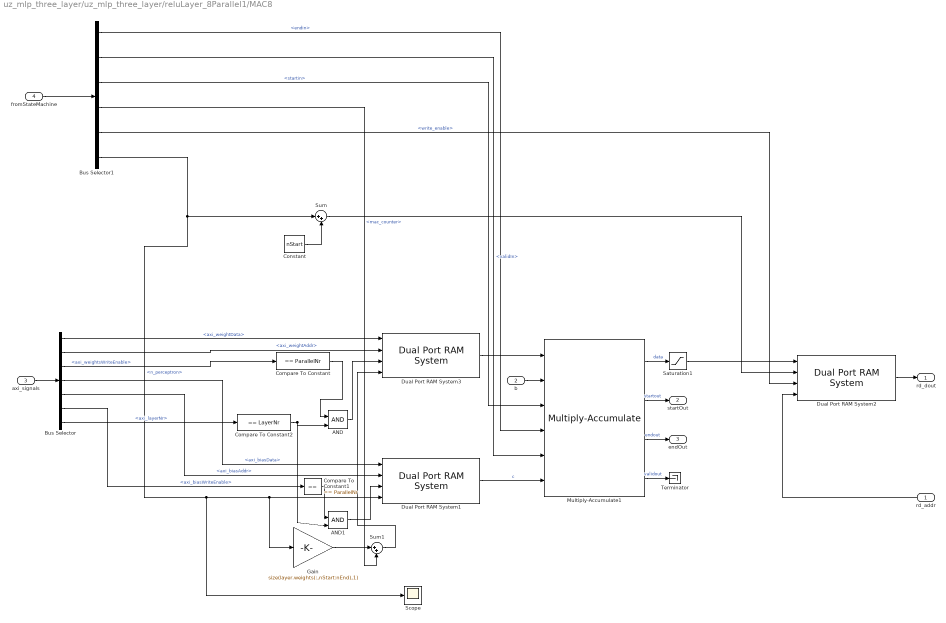
== system uz_mlp_three_layer/uz_mlp_three_layer/reluLayer_8Parallel1/MAC8 ==
  rd_addr : Inport
  b : Inport  Port=2
  axi_signals : Inport  Port=3
  fromStateMachine : Inport  Port=4
  AND : Logic  IconShape=distinctive  AllPortsSameDT=off  OutDataTypeStr=boolean
  AND1 : Logic  IconShape=distinctive  AllPortsSameDT=off  OutDataTypeStr=boolean
  Bus Selector : BusSelector  OutputSignals=axi_weightData,axi_weightAddr,axi_weightsWriteEnable,axi_biasData,axi_biasAddr,axi_biasWriteEnable,axi_layerNr
  Bus Selector1 : BusSelector  OutputSignals=endin,validIn,startin,mac_counter,write_enable,n_perceptron
  Compare To Constant : simulink/Logic and Bit Operations/Compare To Constant  relop===  const=ParallelNr  OutDataTypeStr=boolean
  Compare To Constant1 : simulink/Logic and Bit Operations/Compare To Constant  relop===  const=ParallelNr  OutDataTypeStr=boolean
  Compare To Constant2 : simulink/Logic and Bit Operations/Compare To Constant  relop===  const=LayerNr  OutDataTypeStr=boolean
  Constant : Constant  Value=nStart  OutDataTypeStr=Inherit: Inherit via back propagation  SampleTime=-1
  Dual Port RAM System1 : hdlsllib/HDL RAMs/Dual Port RAM System  RAMType=Simple dual port  WriteOutputValue=New data  RAMInitialValue=[layer.bias(nStart:nEnd);zeros(1024-length(layer.bias(nStart:nEnd)),1)]  SimulateUsing=Code generation
      settings: SourceProductBaseCode=SL
  Dual Port RAM System2 : hdlsllib/HDL RAMs/Dual Port RAM System  RAMType=Simple dual port  WriteOutputValue=New data  RAMInitialValue=[0]  SimulateUsing=Code generation
      settings: SourceProductBaseCode=SL
  Dual Port RAM System3 : hdlsllib/HDL RAMs/Dual Port RAM System  RAMType=Simple dual port  WriteOutputValue=New data  RAMInitialValue=[0;reshape(layer.weights(:,nStart:nEnd),[],1);zeros(1023-length(reshape(layer.weights(:,nStart:nEnd),[],1)),1)]  SimulateUsing=Code generation
      settings: SourceProductBaseCode=SL
  Gain : Gain  Gain=size(layer.weights(:,nStart:nEnd),1)  OutDataTypeStr=Inherit: Same as input
  Multiply-Accumulate1 : hdlsllib/HDL Operations/Multiply-Accumulate  opMode=Streaming - using Start and End ports  initValueSetting=Dialog  initValue=0  initValueSetting2=Input port  initValue2=0  initValueSetting3=Dialog  initValue3=0  num_samples=2  RndMeth2=Floor  RndMeth3=Floor  datatype2=fixdt(1,32,14)  datatype3=Inherit: Inherit via back propagation  validOut=on  endInandOut=on  startOut=on  countOut=on  dim=-1  DoSatur=off  parallel=off
      settings: SourceProductBaseCode=SL
  Saturation1 : Saturate  UpperLimit=nn_data_type_max  LowerLimit=0
  Scope : Scope
  Sum : Sum  Inputs=|++  OutDataTypeStr=Inherit: Same as first input
  Sum1 : Sum  Inputs=|++  OutDataTypeStr=Inherit: Same as first input
  Terminator : Terminator
  rd_dout : Outport
  startOut : Outport  Port=2
  endOut : Outport  Port=3
  wires:
  Dual Port RAM System1/1 -> Multiply-Accumulate1/6  "c"
  Saturation1/1 -> Dual Port RAM System2/1
  Multiply-Accumulate1/4 -> Terminator/1  "validout"
  Multiply-Accumulate1/2 -> startOut/1  "startout"
  Multiply-Accumulate1/1 -> Saturation1/1  "data"
  b/1 -> Multiply-Accumulate1/2
  Bus Selector1/6 -> Sum/1, Gain/1, Dual Port RAM System1/4, Scope/1  "<n_perceptron>"
  Constant/1 -> Sum/2
  Bus Selector1/1 -> Multiply-Accumulate1/4  "<endin>"
  Multiply-Accumulate1/3 -> endOut/1  "endout"
  Dual Port RAM System2/1 -> rd_dout/1
  Bus Selector1/4 -> Sum1/2  "<mac_counter>"
  Bus Selector1/2 -> Multiply-Accumulate1/5  "<validIn>"
  Bus Selector1/3 -> Multiply-Accumulate1/3  "<startin>"
  Gain/1 -> Sum1/1
  Sum1/1 -> Dual Port RAM System3/4
  Sum/1 -> Dual Port RAM System2/2
  Bus Selector1/5 -> Dual Port RAM System2/3  "<write_enable>"
  rd_addr/1 -> Dual Port RAM System2/4
  Dual Port RAM System3/1 -> Multiply-Accumulate1/1
  Bus Selector/4 -> Dual Port RAM System1/1  "<axi_biasData>"
  Bus Selector/5 -> Dual Port RAM System1/2  "<axi_biasAddr>"
  Bus Selector/6 -> Compare To Constant1/1  "<axi_biasWriteEnable>"
  Bus Selector/1 -> Dual Port RAM System3/1  "<axi_weightData>"
  Bus Selector/2 -> Dual Port RAM System3/2  "<axi_weightAddr>"
  Bus Selector/3 -> Compare To Constant/1  "<axi_weightsWriteEnable>"
  axi_signals/1 -> Bus Selector/1
  Compare To Constant/1 -> AND/1
  Compare To Constant1/1 -> AND1/1
  Compare To Constant2/1 -> AND1/2, AND/2
  AND/1 -> Dual Port RAM System3/3
  Bus Selector/7 -> Compare To Constant2/1  "<axi_layerNr>"
  AND1/1 -> Dual Port RAM System1/3
  fromStateMachine/1 -> Bus Selector1/1

== system uz_mlp_three_layer/uz_mlp_three_layer/LastLayer/parallelOutput/holdValue ==
  note: Outputs data if "takeNewValue" is 1
      | Otherwise, outputs the last value of data when takeNewValue was 1
  takeNewValue : Inport
  data : Inport  Port=2
  Delay1 : Delay  DelayLength=1
  Switch : Switch  Criteria=u2 ~= 0
  out : Outport
  wires:
  Switch/1 -> out/1, Delay1/1
  takeNewValue/1 -> Switch/2
  Delay1/1 -> Switch/3
  data/1 -> Switch/1

== system uz_mlp_three_layer/uz_mlp_three_layer/LastLayer/parallelOutput/holdValue1 ==
  note: Outputs data if "takeNewValue" is 1
      | Otherwise, outputs the last value of data when takeNewValue was 1
  takeNewValue : Inport
  data : Inport  Port=2
  Delay1 : Delay  DelayLength=1
  Switch : Switch  Criteria=u2 ~= 0
  out : Outport
  wires:
  Switch/1 -> out/1, Delay1/1
  takeNewValue/1 -> Switch/2
  Delay1/1 -> Switch/3
  data/1 -> Switch/1

== system uz_mlp_three_layer/uz_mlp_three_layer/LastLayer/parallelOutput/holdValue2 ==
  note: Outputs data if "takeNewValue" is 1
      | Otherwise, outputs the last value of data when takeNewValue was 1
  takeNewValue : Inport
  data : Inport  Port=2
  Delay1 : Delay  DelayLength=1
  Switch : Switch  Criteria=u2 ~= 0
  out : Outport
  wires:
  Switch/1 -> out/1, Delay1/1
  takeNewValue/1 -> Switch/2
  Delay1/1 -> Switch/3
  data/1 -> Switch/1

== system uz_mlp_three_layer/uz_mlp_three_layer/LastLayer/parallelOutput/holdValue3 ==
  note: Outputs data if "takeNewValue" is 1
      | Otherwise, outputs the last value of data when takeNewValue was 1
  takeNewValue : Inport
  data : Inport  Port=2
  Delay1 : Delay  DelayLength=1
  Switch : Switch  Criteria=u2 ~= 0
  out : Outport
  wires:
  Switch/1 -> out/1, Delay1/1
  takeNewValue/1 -> Switch/2
  Delay1/1 -> Switch/3
  data/1 -> Switch/1

== system uz_mlp_three_layer/uz_mlp_three_layer/LastLayer/parallelOutput/holdValue4 ==
  note: Outputs data if "takeNewValue" is 1
      | Otherwise, outputs the last value of data when takeNewValue was 1
  takeNewValue : Inport
  data : Inport  Port=2
  Delay1 : Delay  DelayLength=1
  Switch : Switch  Criteria=u2 ~= 0
  out : Outport
  wires:
  Switch/1 -> out/1, Delay1/1
  takeNewValue/1 -> Switch/2
  Delay1/1 -> Switch/3
  data/1 -> Switch/1

== system uz_mlp_three_layer/uz_mlp_three_layer/LastLayer/parallelOutput/holdValue5 ==
  note: Outputs data if "takeNewValue" is 1
      | Otherwise, outputs the last value of data when takeNewValue was 1
  takeNewValue : Inport
  data : Inport  Port=2
  Delay1 : Delay  DelayLength=1
  Switch : Switch  Criteria=u2 ~= 0
  out : Outport
  wires:
  Switch/1 -> out/1, Delay1/1
  takeNewValue/1 -> Switch/2
  Delay1/1 -> Switch/3
  data/1 -> Switch/1

== system uz_mlp_three_layer/uz_mlp_three_layer/LastLayer/parallelOutput/holdValue6 ==
  note: Outputs data if "takeNewValue" is 1
      | Otherwise, outputs the last value of data when takeNewValue was 1
  takeNewValue : Inport
  data : Inport  Port=2
  Delay1 : Delay  DelayLength=1
  Switch : Switch  Criteria=u2 ~= 0
  out : Outport
  wires:
  Switch/1 -> out/1, Delay1/1
  takeNewValue/1 -> Switch/2
  Delay1/1 -> Switch/3
  data/1 -> Switch/1

== system uz_mlp_three_layer/uz_mlp_three_layer/LastLayer/parallelOutput/holdValue7 ==
  note: Outputs data if "takeNewValue" is 1
      | Otherwise, outputs the last value of data when takeNewValue was 1
  takeNewValue : Inport
  data : Inport  Port=2
  Delay1 : Delay  DelayLength=1
  Switch : Switch  Criteria=u2 ~= 0
  out : Outport
  wires:
  Switch/1 -> out/1, Delay1/1
  takeNewValue/1 -> Switch/2
  Delay1/1 -> Switch/3
  data/1 -> Switch/1

== stateflow chart uz_mlp_three_layer/reluLayer_4Parallel/StateMachines1/mac_control ==
  settings: executeAtInitialization=1
  state idle_entry
    index_counter_rst=true;
    index_counter_enb=false;
    mac_startIn=false;
    mac_endIn=false;
    mac_validIn=false;
    mac_ready=true;
    write_ram=false;
  state start_counter
    index_counter_rst=false;
    index_counter_enb=true;
    mac_ready=false;
  state write_ram_entry
    write_ram=true;
  state start_mac
    mac_startIn=true;
    mac_validIn=true;
  state accumulate
    mac_startIn=false;
  state mac_stop
    mac_endIn=false;
    mac_validIn=false;
    index_counter_rst=true;
    index_counter_enb=false;
  state mac_finished
    mac_endIn=true;
  (default) -> idle_entry
  idle_entry -> start_counter : [external_enable==true]
  write_ram_entry -> idle_entry
  start_counter -> start_mac
  mac_stop -> write_ram_entry : [end_out_delay==true]
  start_mac -> accumulate : [mac_startOut==true]
  accumulate -> mac_finished : [counter_finished==true]
  mac_finished -> mac_stop : [end_out==true]
  data: index_counter_enb output boolean; mac_startIn output boolean; mac_endIn output boolean; mac_validIn output boolean; index_counter_rst output boolean; external_enable input boolean; counter_finished input boolean; end_out input boolean; end_out_delay input boolean; write_ram output boolean; mac_startOut input boolean; mac_ready output boolean

== stateflow chart uz_mlp_three_layer/LastLayer/StateMachines/layer_control ==
  settings: executeAtInitialization=1
  state entry_to_entry_state
    layer_rdy=true;
    counter_rest=true; % reset counter for looping through perceptrons of one layer
  state calc_perceptron
    enable_mac=true;
  state idle
    cnt_enable=false;
  state finished2
    layer_finished=false;
  state perceptron_rdy
    cnt_enable=true;
    counter_rest=false;
  state finished
    layer_finished=true;
  state calc_running
    enable_mac=false;
  (default) -> entry_to_entry_state
  finished2 -> entry_to_entry_state
  entry_to_entry_state -> idle : [ext_enable==true]
  idle -> calc_perceptron : [mac_ready==true ]
  calc_perceptron -> calc_running : [mac_ready==false]
  perceptron_rdy -> idle
  finished -> finished2
  calc_running -> perceptron_rdy [order 1] : [mac_ready==true && cnt_finished==false]
  calc_running -> finished [order 2] : [mac_ready==true & cnt_finished==true]
  data: ext_enable input boolean; enable_mac output boolean; mac_ready input boolean; layer_rdy output boolean; cnt_enable output boolean; counter_rest output boolean; cnt_finished input boolean; layer_finished output

== stateflow chart uz_mlp_three_layer/LastLayer/StateMachines/mac_control ==
  settings: executeAtInitialization=1
  state idle_entry
    index_counter_rst=true;
    index_counter_enb=false;
    mac_startIn=false;
    mac_endIn=false;
    mac_validIn=false;
    mac_ready=true;
    write_ram=false;
  state start_counter
    index_counter_rst=false;
    index_counter_enb=true;
    mac_ready=false;
  state write_ram_entry
    write_ram=true;
  state start_mac
    mac_startIn=true;
    mac_validIn=true;
  state accumulate
    mac_startIn=false;
  state mac_stop
    mac_endIn=false;
    mac_validIn=false;
    index_counter_rst=true;
    index_counter_enb=false;
  state mac_finished
    mac_endIn=true;
  (default) -> idle_entry
  idle_entry -> start_counter : [external_enable==true]
  write_ram_entry -> idle_entry
  start_counter -> start_mac
  mac_stop -> write_ram_entry : [end_out_delay==true]
  start_mac -> accumulate : [mac_startOut==true]
  accumulate -> mac_finished : [counter_finished==true]
  mac_finished -> mac_stop : [end_out==true]
  data: index_counter_enb output boolean; mac_startIn output boolean; mac_endIn output boolean; mac_validIn output boolean; index_counter_rst output boolean; external_enable input boolean; counter_finished input boolean; end_out input boolean; end_out_delay input boolean; write_ram output boolean; mac_startOut input boolean; mac_ready output boolean

== matlab function uz_mlp_three_layer/reluLayer_8Parallel1/MATLAB Function1 ==
  settings: fimath=fimath('RoundingMethod', 'Floor','OverflowAction', 'Wrap','ProductMode', 'FullPrecision', 'SumMode', 'FullPrecision')
  data: readAddr input; y output
function y = fcn(readAddr)

y=uint8(0);
if (readAddr>0 && readAddr <= 8)
    y=uint8(0);
end
if (readAddr>8 && readAddr <= 16)
    y=uint8(1);
end
if (readAddr>16 && readAddr <= 24)
    y=uint8(2);
end
if (readAddr>24 && readAddr <= 32)
    y=uint8(3);
end
if (readAddr>32 && readAddr <= 40)
    y=uint8(4);
end
if (readAddr>40 && readAddr <= 48)
    y=uint8(5);
end
if (readAddr>48 && readAddr <= 56)
    y=uint8(6);
end
if (readAddr>56 && readAddr <= 64)
    y=uint8(7);
end

== matlab function uz_mlp_three_layer/reluLayer_8Parallel/MATLAB Function1 ==
  settings: fimath=fimath('RoundingMethod', 'Floor','OverflowAction', 'Wrap','ProductMode', 'FullPrecision', 'SumMode', 'FullPrecision')
  data: readAddr input; y output
function y = fcn(readAddr)

y=uint8(0);
if (readAddr>0 && readAddr <= 8)
    y=uint8(0);
end
if (readAddr>8 && readAddr <= 16)
    y=uint8(1);
end
if (readAddr>16 && readAddr <= 24)
    y=uint8(2);
end
if (readAddr>24 && readAddr <= 32)
    y=uint8(3);
end
if (readAddr>32 && readAddr <= 40)
    y=uint8(4);
end
if (readAddr>40 && readAddr <= 48)
    y=uint8(5);
end
if (readAddr>48 && readAddr <= 56)
    y=uint8(6);
end
if (readAddr>56 && readAddr <= 64)
    y=uint8(7);
end

== matlab function uz_mlp_three_layer/reluLayer_4Parallel/MATLAB Function ==
  settings: fimath=fimath('RoundingMethod', 'Floor','OverflowAction', 'Wrap','ProductMode', 'FullPrecision', 'SumMode', 'FullPrecision')
  data: readAddr input; y output
function y = fcn(readAddr)

y=uint8(0);
if (readAddr>0 && readAddr <= 16)
    y=uint8(0);
end
if (readAddr>16 && readAddr <= 32)
    y=uint8(1);
end
if (readAddr>32 && readAddr <= 48)
    y=uint8(2);
end
if (readAddr>48 && readAddr <= 64)
    y=uint8(3);
end
